simulink model "codreto"  (R2022b)
settings: Solver=FixedStepAuto  StartTime=0.0  StopTime=inf  RelTol=1e-3
undefined symbols (not defined in the file): hw
libraries: raspberrypiIOTlib x2, raspberrypiAVlib x1, dspspect3 x1, audiofilters x1, dspsigops x1
settings Model: SimulationMode=external  Creator=danar  LastModifiedBy=josaf
settings SolverCC: PositivePriorityOrder=on
settings OptimizationCC: EnhancedBackFolding=on  PassReuseOutputArgsAs=Individual arguments  ZeroExternalMemoryAtStartup=off  ZeroInternalMemoryAtStartup=off  MaxStackSize=64  OptimizeBlockOrder=speed  DifferentSizesBufferReuse=on  OptimizationCustomize=off  EfficientTunableParamExpr=on
settings DebuggingCC: ParameterTunabilityLossMsg=error
settings HardwareCC: ProdBitPerPointer=32  ProdBitPerSizeT=32  ProdBitPerPtrDiffT=32  ProdLargestAtomicInteger=Long  ProdLargestAtomicFloat=Double  ProdWordSize=32  ProdLongLongMode=on  ProdHWDeviceType=ARM Compatible->ARM Cortex  UseEmbeddedCoderFeatures=off  UseSimulinkCoderFeatures=off
settings ModelReferenceCC: EnableRefExpFcnMdlSchedulingChecks=on
settings RTWCC: Description=Embedded Coder  SystemTargetFile=ert.tlc  HardwareBoard=Raspberry Pi  TemplateMakefile=ert_default_tmf  RTWVerbose=off  Toolchain=GNU GCC Embedded Linux  BuildConfiguration=Faster Runs
settings CodeAppCC: ForceParamTrailComments=on  OperatorAnnotations=on  SimulinkDataObjDesc=on  SFDataObjDesc=on  MangleLength=10  InsertBlockDesc=on
settings ERTTargetCC: SupportNonInlinedSFcns=on  SupportVariableSizeSignals=on  ExtMode=on  ExtModeTransport=2  ExtModeStaticAlloc=on  ExtModeMexFile=ext_xcp  ExtModeMexArgs='10.50.90.39' 0 17725  ExtModeIntrfLevel=Level2 - Open  ERTSrcFileBannerTemplate=codertarget_code_template.cgt  ERTHdrFileBannerTemplate=codertarget_code_template.cgt  ERTDataSrcFileTemplate=codertarget_code_template.cgt  ERTDataHdrFileTemplate=codertarget_code_template.cgt

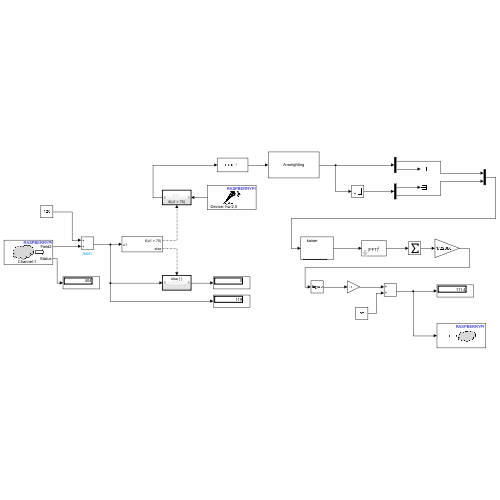
[thumbnail: Simulink's stored preview of the top-level diagram]
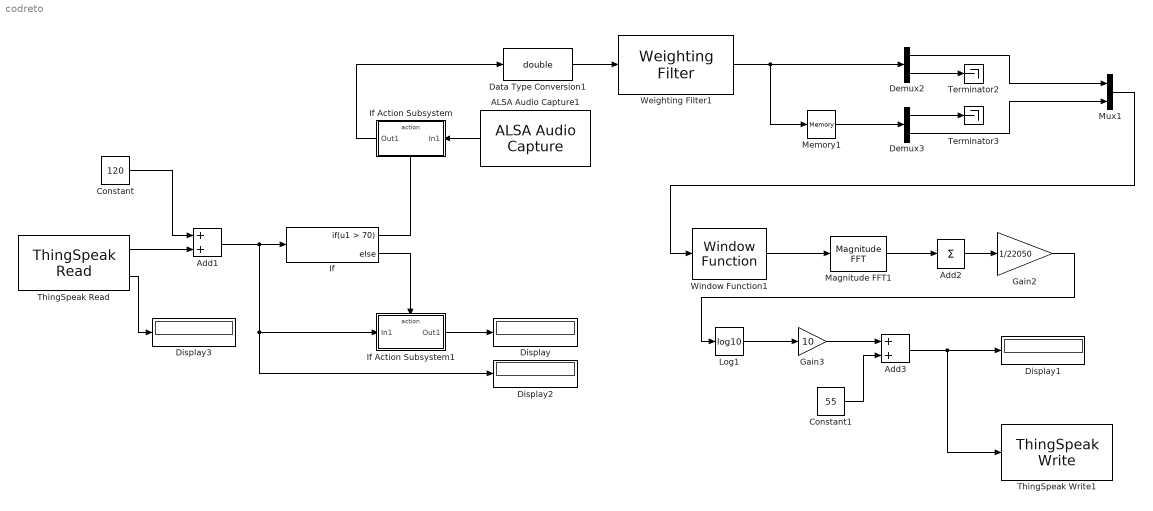
== system codreto ==
  ALSA Audio Capture1 : raspberrypiAVlib/ALSA Audio Capture  deviceStr=hw:2,0  DataBitDepth=16-bit integer  numberOfChannels=1  sampleRateEnum=44100  frameSize=22050  QueueDuration=0.5  blockPlatform=LINUX
  Add1 : Sum
  Add2 : Sum  Inputs=+
  Add3 : Sum
  Constant : Constant  Value=120
  Constant1 : Constant  Value=55
  Data Type Conversion1 : DataTypeConversion  OutDataTypeStr=double  RndMeth=Nearest
  Demux2 : Demux  Outputs=2
  Demux3 : Demux  Outputs=2
  Display{,1..3} (4 alike) : Display
  Gain2 : Gain  Gain=1/22050
  Gain3 : Gain  Gain=10
  If : If  IfExpression=u1 > 70
  If Action Subsystem : Subsystem  TreatAsAtomicUnit=on
  If Action Subsystem1 : Subsystem  TreatAsAtomicUnit=on
  Log1 : Math  Operator=log10
  Magnitude FFT1 : dspspect3/Magnitude FFT  mag_or_magsq=Magnitude squared  FFTImplementation=Auto  fftLenInherit=off  fftsize=32768  WrapInput=on
  Memory1 : Memory
  Mux1 : Mux  Inputs=2
  Terminator2 : Terminator
  Terminator3 : Terminator
  ThingSpeak Read : raspberrypiIOTlib/ThingSpeak Read  ChannelID=1  ChannelAccess=Private  ReadAPIKey=3ARL9SJHBUQ607AZ  FieldNumber=2  PrintDiagnosticMessages=off  SampleTime=30  blockPlatform=LINUX
  ThingSpeak Write1 : raspberrypiIOTlib/ThingSpeak Write  UpdateURL=https://api.thingspeak.com/update  WriteAPIKey=LE4VKE1LVSEK7ARF  NumberOfFields=1  UpdateInterval=30  PrintDiagnosticMessages=on  CoordinatesEnabled=off  CoordSrc=Block dialog  Coordinates=[42.29971, -71.350719, 69.29]  blockPlatform=Raspberry Pi
  Weighting Filter1 : audiofilters/Weighting Filter  Method=A-weighting  InheritSampleRate=off  SampleRate=44100  SimulateUsing=Code generation  WorkspaceVariableName=myFilt  OverwriteExportVariable=on  MaskClassType=No mask
  Window Function1 : dspsigops/Window Function  winmode=Apply window to input  wintype=Kaiser  sampmode=Continuous  samptime=1  N=5  Rs=50  beta=5  winsamp=Symmetric  UserWindow=hamming  OptParams=off  UserParams={'symmetric'}  dataType=double  isSigned=on  wordLen=16  udDataType=sfix(16)  fracBitsMode=Best precision  numFracBits=15  roundingMode=Floor  overflowMode=off  numSidelobes=4  sidelobeLevel=-30
  wires:
  Data Type Conversion1/1 -> Weighting Filter1/1
  Demux3/1 -> Terminator3/1
  Demux2/2 -> Terminator2/1
  Demux3/2 -> Mux1/2
  Demux2/1 -> Mux1/1
  Memory1/1 -> Demux3/1
  Mux1/1 -> Window Function1/1
  Gain2/1 -> Log1/1
  Add3/1 -> Display1/1, ThingSpeak Write1/1
  Constant1/1 -> Add3/2
  Gain3/1 -> Add3/1
  Log1/1 -> Gain3/1
  Add2/1 -> Gain2/1
  Magnitude FFT1/1 -> Add2/1
  Window Function1/1 -> Magnitude FFT1/1
  Weighting Filter1/1 -> Memory1/1, Demux2/1
  ALSA Audio Capture1/1 -> If Action Subsystem/1(In1)
  If/1 -> If Action Subsystem/Action
  If/2 -> If Action Subsystem1/Action
  If Action Subsystem1/1(Out1) -> Display/1
  If Action Subsystem/1(Out1) -> Data Type Conversion1/1
  ThingSpeak Read/2 -> Display3/1
  ThingSpeak Read/1 -> Add1/2
  Add1/1 -> Display2/1, If Action Subsystem1/1(In1), If/1
  Constant/1 -> Add1/1

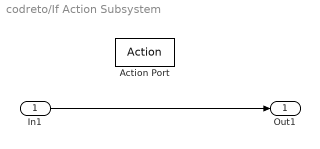
== system codreto/If Action Subsystem ==
  In1 : Inport
  Action Port : ActionPort  ActionPortLabel=if(u1 > 70)
  Out1 : Outport
  wires:
  In1/1 -> Out1/1

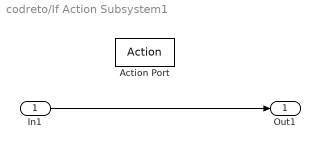
== system codreto/If Action Subsystem1 ==
  In1 : Inport
  Action Port : ActionPort  ActionPortLabel=else
  Out1 : Outport
  wires:
  In1/1 -> Out1/1
